simulink model "ME190project1"  (R2017a)
settings: Solver=ode5  StartTime=0.0  StopTime=1  FixedStep=0.001  RelTol=1e-3
values from neighbouring files (symbols this model uses):
  A = [zeros(2) eye(2); -inv(M)*K -inv(M)*D]    [project1mat.m]
  B = [0; 0; inv(M)*F]    [project1mat.m]
  C = eye(4)    [project1mat.m]
  DS = [0 0 0 0]'    [project1mat.m]
  IN = [0;(n*3.14/180);0;0]    [project1mat.m]
settings Model: Creator=kiran  LastModifiedBy=kiran

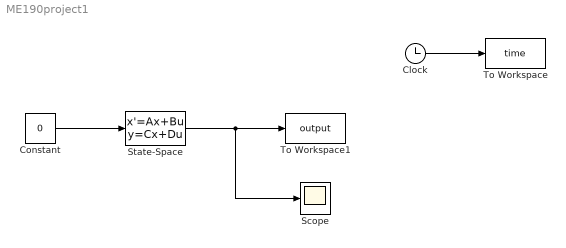
== system ME190project1 ==
  Clock : Clock
  Constant : Constant  Value=0
  Scope : Scope
  State-Space : StateSpace  A=A  B=B  C=C  D=DS  X0=IN
  To Workspace : ToWorkspace  VariableName=time  SampleTime=-1
  To Workspace1 : ToWorkspace  VariableName=output  SampleTime=-1
  wires:
  Clock/1 -> To Workspace/1
  State-Space/1 -> Scope/1, To Workspace1/1
  Constant/1 -> State-Space/1
